simulink model "calcDesTanRollAng_th"  (R2020a)
settings: Solver=VariableStepAuto  StartTime=0.0  StopTime=10.0  RelTol=1e-3
undefined symbols (not defined in the file or in its folder): f_kitePos, f_kiteVel, kiteMass, maxTanRoll_deg, netWingLift, rTarget, turnAng
libraries: calcDesTanRollAng_ul x1
settings Model: Creator=Ayaz  LastModifiedBy=Ayaz

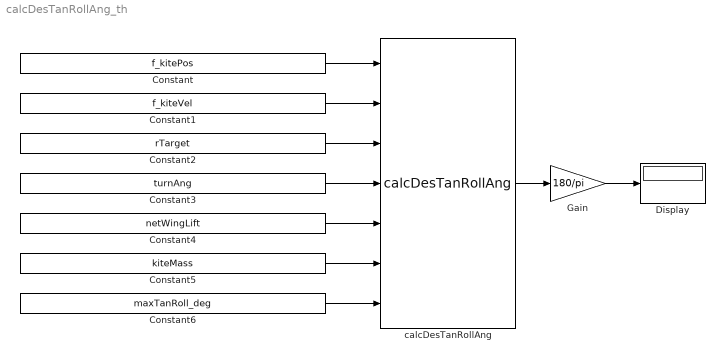
== system calcDesTanRollAng_th ==
  Constant : Constant  Value=f_kitePos  VectorParams1D=off
  Constant1 : Constant  Value=f_kiteVel  VectorParams1D=off
  Constant2 : Constant  Value=rTarget  VectorParams1D=off
  Constant3 : Constant  Value=turnAng
  Constant4 : Constant  Value=netWingLift
  Constant5 : Constant  Value=kiteMass
  Constant6 : Constant  Value=maxTanRoll_deg
  Display : Display
  Gain : Gain  Gain=180/pi
  calcDesTanRollAng : calcDesTanRollAng_ul/calcDesTanRollAng  SystemSampleTime=-1  Latency=0  AutoFrameSizeCalculation=off
  wires:
  Constant/1 -> calcDesTanRollAng/1
  Constant1/1 -> calcDesTanRollAng/2
  Constant2/1 -> calcDesTanRollAng/3
  Constant3/1 -> calcDesTanRollAng/4
  Constant4/1 -> calcDesTanRollAng/5
  Constant5/1 -> calcDesTanRollAng/6
  Constant6/1 -> calcDesTanRollAng/7
  calcDesTanRollAng/1 -> Gain/1
  Gain/1 -> Display/1
